simulink model "EGRVlv"  (R2018a)
settings: configuration reference "cs_ert" (kept outside this file)
settings Model: DataDictionary=EGRVlv.sldd  Creator=zhoutinglin  LastModifiedBy=zhoutinglin

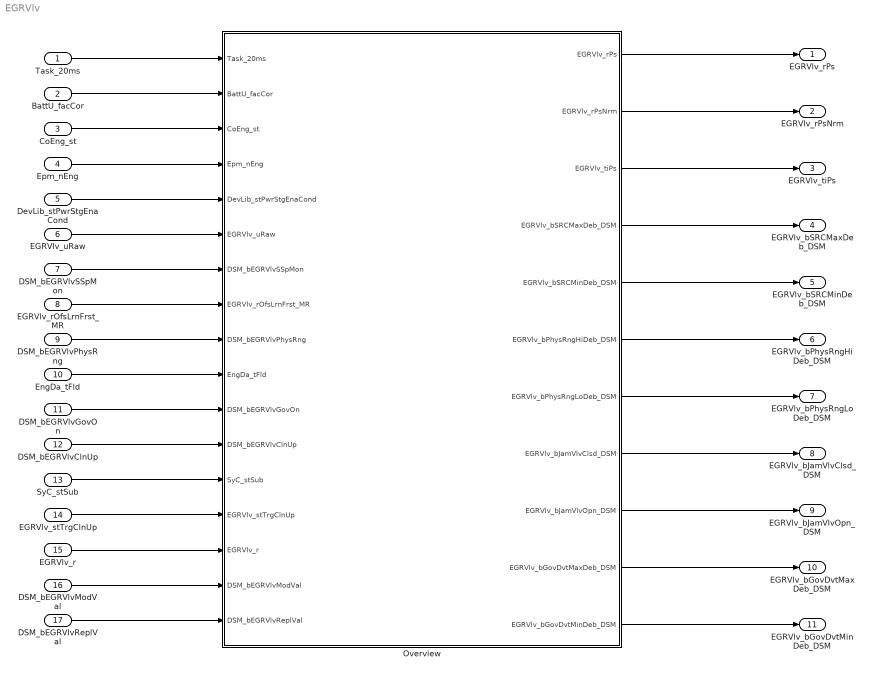
== system EGRVlv ==
  Task_20ms : Inport  SampleTime=20  OutputFunctionCall=on
  BattU_facCor : Inport  Port=2
  CoEng_st : Inport  Port=3
  Epm_nEng : Inport  Port=4
  DevLib_stPwrStgEnaCond : Inport  Port=5
  EGRVlv_uRaw : Inport  Port=6
  DSM_bEGRVlvSSpMon : Inport  Port=7
  EGRVlv_rOfsLrnFrst_MR : Inport  Port=8
  DSM_bEGRVlvPhysRng : Inport  Port=9
  EngDa_tFld : Inport  Port=10
  DSM_bEGRVlvGovOn : Inport  Port=11
  DSM_bEGRVlvClnUp : Inport  Port=12
  SyC_stSub : Inport  Port=13
  EGRVlv_stTrgClnUp : Inport  Port=14
  EGRVlv_r : Inport  Port=15
  DSM_bEGRVlvModVal : Inport  Port=16
  DSM_bEGRVlvReplVal : Inport  Port=17
  Overview : Subsystem
  EGRVlv_rPs : Outport
  EGRVlv_rPsNrm : Outport  Port=2
  EGRVlv_tiPs : Outport  Port=3
  EGRVlv_bSRCMaxDeb_DSM : Outport  Port=4
  EGRVlv_bSRCMinDeb_DSM : Outport  Port=5
  EGRVlv_bPhysRngHiDeb_DSM : Outport  Port=6
  EGRVlv_bPhysRngLoDeb_DSM : Outport  Port=7
  EGRVlv_bJamVlvClsd_DSM : Outport  Port=8
  EGRVlv_bJamVlvOpn_DSM : Outport  Port=9
  EGRVlv_bGovDvtMaxDeb_DSM : Outport  Port=10
  EGRVlv_bGovDvtMinDeb_DSM : Outport  Port=11
  wires:
  BattU_facCor/1 -> Overview/2(BattU_facCor)
  CoEng_st/1 -> Overview/3(CoEng_st)
  Epm_nEng/1 -> Overview/4(Epm_nEng)
  DevLib_stPwrStgEnaCond/1 -> Overview/5(DevLib_stPwrStgEnaCond)
  EGRVlv_uRaw/1 -> Overview/6(EGRVlv_uRaw)
  DSM_bEGRVlvSSpMon/1 -> Overview/7(DSM_bEGRVlvSSpMon)
  EGRVlv_rOfsLrnFrst_MR/1 -> Overview/8(EGRVlv_rOfsLrnFrst_MR)
  DSM_bEGRVlvPhysRng/1 -> Overview/9(DSM_bEGRVlvPhysRng)
  EngDa_tFld/1 -> Overview/10(EngDa_tFld)
  DSM_bEGRVlvGovOn/1 -> Overview/11(DSM_bEGRVlvGovOn)
  DSM_bEGRVlvClnUp/1 -> Overview/12(DSM_bEGRVlvClnUp)
  SyC_stSub/1 -> Overview/13(SyC_stSub)
  EGRVlv_stTrgClnUp/1 -> Overview/14(EGRVlv_stTrgClnUp)
  EGRVlv_r/1 -> Overview/15(EGRVlv_r)
  DSM_bEGRVlvModVal/1 -> Overview/16(DSM_bEGRVlvModVal)
  DSM_bEGRVlvReplVal/1 -> Overview/17(DSM_bEGRVlvReplVal)
  Task_20ms/1 -> Overview/1(Task_20ms)
  Overview/1(EGRVlv_rPs) -> EGRVlv_rPs/1
  Overview/2(EGRVlv_rPsNrm) -> EGRVlv_rPsNrm/1
  Overview/3(EGRVlv_tiPs) -> EGRVlv_tiPs/1
  Overview/4(EGRVlv_bSRCMaxDeb_DSM) -> EGRVlv_bSRCMaxDeb_DSM/1
  Overview/5(EGRVlv_bSRCMinDeb_DSM) -> EGRVlv_bSRCMinDeb_DSM/1
  Overview/6(EGRVlv_bPhysRngHiDeb_DSM) -> EGRVlv_bPhysRngHiDeb_DSM/1
  Overview/7(EGRVlv_bPhysRngLoDeb_DSM) -> EGRVlv_bPhysRngLoDeb_DSM/1
  Overview/8(EGRVlv_bJamVlvClsd_DSM) -> EGRVlv_bJamVlvClsd_DSM/1
  Overview/9(EGRVlv_bJamVlvOpn_DSM) -> EGRVlv_bJamVlvOpn_DSM/1
  Overview/10(EGRVlv_bGovDvtMaxDeb_DSM) -> EGRVlv_bGovDvtMaxDeb_DSM/1
  Overview/11(EGRVlv_bGovDvtMinDeb_DSM) -> EGRVlv_bGovDvtMinDeb_DSM/1

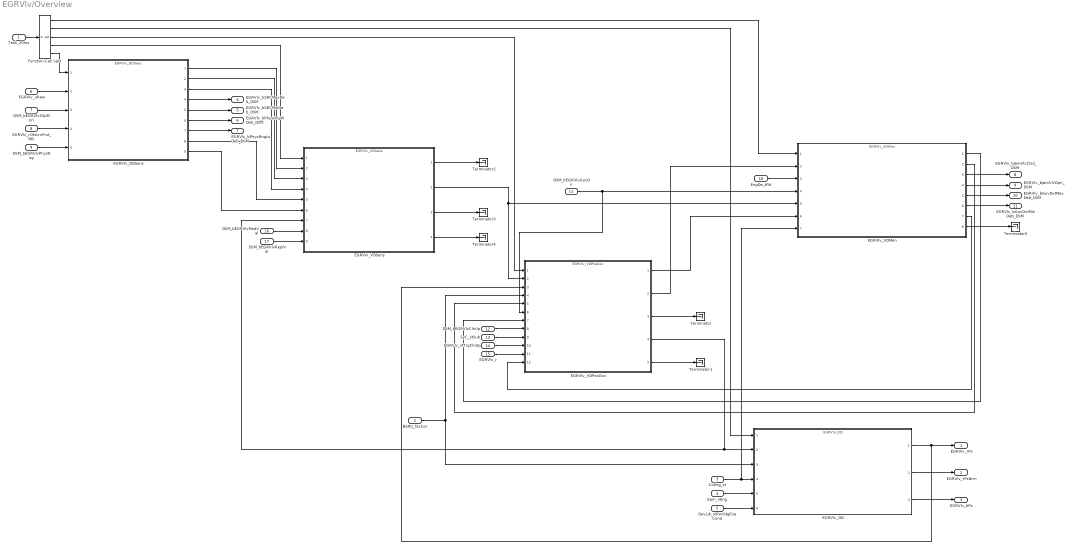
== system EGRVlv/Overview ==
  Task_20ms : Inport
  BattU_facCor : Inport  Port=2
  CoEng_st : Inport  Port=3
  Epm_nEng : Inport  Port=4
  DevLib_stPwrStgEnaCond : Inport  Port=5
  EGRVlv_uRaw : Inport  Port=6
  DSM_bEGRVlvSSpMon : Inport  Port=7
  EGRVlv_rOfsLrnFrst_MR : Inport  Port=8
  DSM_bEGRVlvPhysRng : Inport  Port=9
  EngDa_tFld : Inport  Port=10
  DSM_bEGRVlvGovOn : Inport  Port=11
  DSM_bEGRVlvClnUp : Inport  Port=12
  SyC_stSub : Inport  Port=13
  EGRVlv_stTrgClnUp : Inport  Port=14
  EGRVlv_r : Inport  Port=15
  DSM_bEGRVlvModVal : Inport  Port=16
  DSM_bEGRVlvReplVal : Inport  Port=17
  EGRVlv_DD : ModelReference  ModelNameDialog=EGRVlv_DD  SimulationMode=Normal  ModelReferenceVersion=1.67
  EGRVlv_DDSens : ModelReference  ModelNameDialog=EGRVlv_DDSens  SimulationMode=Normal  ModelReferenceVersion=1.60
  EGRVlv_VDMon : ModelReference  ModelNameDialog=EGRVlv_VDMon  SimulationMode=Normal  ModelReferenceVersion=1.69
  EGRVlv_VDPosGov : ModelReference  ModelNameDialog=EGRVlv_VDPosGov  SimulationMode=Normal  ModelReferenceVersion=1.82
  EGRVlv_VDSens : ModelReference  ModelNameDialog=EGRVlv_VDSens  SimulationMode=Normal  ModelReferenceVersion=1.67
  Function-Call Split : FunctionCallSplit  IconShape=distinctive  NumOutputPorts=5  OutputPortLayout=default
  Terminator{,1..5} (6 alike) : Terminator
  EGRVlv_rPs : Outport
  EGRVlv_rPsNrm : Outport  Port=2
  EGRVlv_tiPs : Outport  Port=3
  EGRVlv_bSRCMaxDeb_DSM : Outport  Port=4
  EGRVlv_bSRCMinDeb_DSM : Outport  Port=5
  EGRVlv_bPhysRngHiDeb_DSM : Outport  Port=6
  EGRVlv_bPhysRngLoDeb_DSM : Outport  Port=7
  EGRVlv_bJamVlvClsd_DSM : Outport  Port=8
  EGRVlv_bJamVlvOpn_DSM : Outport  Port=9
  EGRVlv_bGovDvtMaxDeb_DSM : Outport  Port=10
  EGRVlv_bGovDvtMinDeb_DSM : Outport  Port=11
  wires:
  EGRVlv_DD/2 -> EGRVlv_rPsNrm/1
  EGRVlv_VDMon/8 -> Terminator5/1
  BattU_facCor/1 -> EGRVlv_VDPosGov/4, EGRVlv_DD/3
  CoEng_st/1 -> EGRVlv_VDMon/7, EGRVlv_DD/4
  Epm_nEng/1 -> EGRVlv_DD/5
  DevLib_stPwrStgEnaCond/1 -> EGRVlv_DD/6
  EGRVlv_DD/3 -> EGRVlv_tiPs/1
  EGRVlv_uRaw/1 -> EGRVlv_DDSens/2
  DSM_bEGRVlvSSpMon/1 -> EGRVlv_DDSens/3
  EGRVlv_rOfsLrnFrst_MR/1 -> EGRVlv_DDSens/4
  DSM_bEGRVlvPhysRng/1 -> EGRVlv_DDSens/5
  EGRVlv_DDSens/1 -> EGRVlv_VDSens/2
  EGRVlv_DDSens/2 -> EGRVlv_VDSens/3
  EGRVlv_DDSens/3 -> EGRVlv_VDSens/4
  EGRVlv_DDSens/4 -> EGRVlv_bSRCMaxDeb_DSM/1
  EGRVlv_DDSens/5 -> EGRVlv_bSRCMinDeb_DSM/1
  EGRVlv_DDSens/6 -> EGRVlv_bPhysRngHiDeb_DSM/1
  EGRVlv_DDSens/7 -> EGRVlv_bPhysRngLoDeb_DSM/1
  EGRVlv_DDSens/8 -> EGRVlv_VDSens/5
  EGRVlv_DDSens/9 -> EGRVlv_VDSens/6
  EngDa_tFld/1 -> EGRVlv_VDMon/3
  DSM_bEGRVlvGovOn/1 -> EGRVlv_VDPosGov/6, EGRVlv_VDMon/4
  EGRVlv_VDMon/3 -> EGRVlv_bJamVlvClsd_DSM/1
  EGRVlv_VDMon/4 -> EGRVlv_bJamVlvOpn_DSM/1
  EGRVlv_VDMon/5 -> EGRVlv_bGovDvtMaxDeb_DSM/1
  EGRVlv_VDMon/6 -> EGRVlv_bGovDvtMinDeb_DSM/1
  DSM_bEGRVlvClnUp/1 -> EGRVlv_VDPosGov/8
  SyC_stSub/1 -> EGRVlv_VDPosGov/9
  EGRVlv_stTrgClnUp/1 -> EGRVlv_VDPosGov/10
  EGRVlv_r/1 -> EGRVlv_VDPosGov/11
  EGRVlv_VDPosGov/1 -> EGRVlv_VDMon/6
  EGRVlv_VDPosGov/2 -> EGRVlv_VDMon/2
  EGRVlv_VDPosGov/3 -> Terminator/1
  EGRVlv_VDPosGov/5 -> Terminator1/1
  DSM_bEGRVlvModVal/1 -> EGRVlv_VDSens/8
  DSM_bEGRVlvReplVal/1 -> EGRVlv_VDSens/9
  EGRVlv_VDSens/1 -> Terminator2/1
  EGRVlv_VDSens/2 -> EGRVlv_VDMon/5, EGRVlv_VDPosGov/2
  EGRVlv_VDSens/3 -> Terminator3/1
  EGRVlv_VDSens/4 -> Terminator4/1
  Task_20ms/1 -> Function-Call Split/1
  Function-Call Split/5 -> EGRVlv_DDSens/1
  Function-Call Split/4 -> EGRVlv_VDSens/1
  Function-Call Split/3 -> EGRVlv_VDPosGov/1
  Function-Call Split/2 -> EGRVlv_DD/1
  Function-Call Split/1 -> EGRVlv_VDMon/1
  EGRVlv_VDMon/7 -> EGRVlv_VDPosGov/12
  EGRVlv_VDMon/1 -> EGRVlv_VDPosGov/7
  EGRVlv_VDMon/2 -> EGRVlv_VDPosGov/5
  EGRVlv_DD/1 -> EGRVlv_VDPosGov/3, EGRVlv_rPs/1
  EGRVlv_VDPosGov/4 -> EGRVlv_VDSens/7, EGRVlv_DD/2
